simulink model "modelo_experimental"  (R2018a)
settings: Solver=VariableStepAuto  StartTime=0.0  StopTime=1  FixedStep=1e-6  MaxStep=1e-4  RelTol=1e-3
PreLoadFcn:
  | SimulinkInit
InitFcn:
  | SimulinkInit
values from neighbouring files (symbols this model uses):
  C1 = 22e-6    (= 2.2e-05)    [SimulinkInit.m]
  C2 = 22e-6    (= 2.2e-05)    [SimulinkInit.m]
  L1 = 40e-3    (= 0.04)    [SimulinkInit.m]
  L2 = 30e-3    (= 0.03)    [SimulinkInit.m]
  L4 = 315e-3    (= 0.315)    [SimulinkInit.m]
  L5 = 220e-3    (= 0.22)    [SimulinkInit.m]
  L6 = 10e-6    (= 1e-05)    [SimulinkInit.m]
  R1 = 0.1    [SimulinkInit.m]
  R2 = 0.2    [SimulinkInit.m]
  R4 = 5    [SimulinkInit.m]
  R5 = 12    [SimulinkInit.m]
  R6 = 0.001    [SimulinkInit.m]
undefined symbols (not defined in the file or in its folder): Ion, Lithium, sigbuilder_block
libraries: powerlib x48, dsparch4 x12, powerlib_meascontrol x3, electricdrivelib x1
settings Model: Creator=erich  LastModifiedBy=MarioAndres
settings CodeAppCC: StateflowObjectComments=on
settings SimscapeCC: SimscapeNormalizeSystem=off

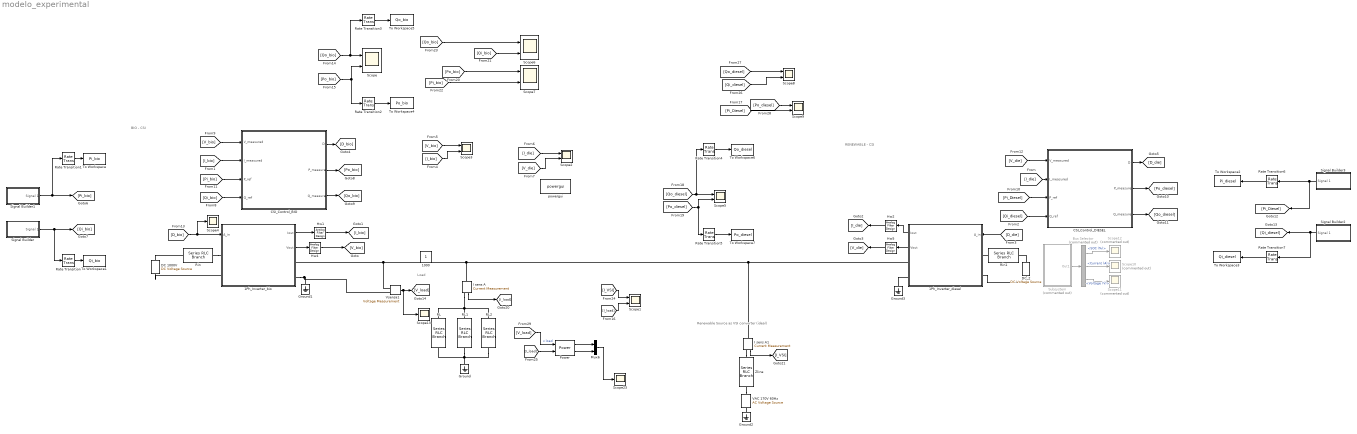
== system modelo_experimental ==
  note: Load
  note: BIO - CSI
  note: RENEWABLE - CSI
  note: Renewable Source as VSI converter (ideal)
  1Ph_Inverter_bio : Subsystem  mask{st_time=0, f_sw=12000, samp_f=1e-6}
      mask prompts: st_time "Tiempo muerto (Start)"; f_sw "Switching frequency"; samp_f "samplig"
      mask Display:
      | port_label('input', 1, 'd', 'texmode', 'on')
      | 
      | port_label('lconn', 1, 'DC +')
      | port_label('lconn', 2, 'DC -')
      | 
      | 
      | port_label('rconn', 1, 'V_{out+}')
      | port_label('rconn', 2, 'B_{out-}')
      | 
      | 
      | port_label('output', 1, 'I_{out}', 'texmode', 'on')
      | port_label('output', 2, 'V_{out}', 'texmode', 'on')
      | 
      | plot([0.1 .9], [0.1 .9])
      | plot([0.2 .4], [.7 .7])
      | plot([0.2 .24], [.65 .65])
      | plot([0.28 .32], [.65 .65])
      | plot([0.36 .40], [.65 .65])
      | 
      | plot([.5:.01:.7], .25+sin(30*[.2:.01:.4])/10)
  1Ph_Inverter_diesel : Subsystem  mask{st_time=0, f_sw=12000, samp_f=1e-6}
      mask prompts: st_time "Tiempo muerto (Start)"; f_sw "Switching frequency"; samp_f "Sampling frequency"
      mask Display:
      | port_label('input', 1, 'd', 'texmode', 'on')
      | 
      | port_label('lconn', 1, 'DC +')
      | port_label('lconn', 2, 'DC -')
      | 
      | 
      | port_label('rconn', 1, 'V_{out+}')
      | port_label('rconn', 2, 'B_{out-}')
      | 
      | 
      | port_label('output', 1, 'I_{out}', 'texmode', 'on')
      | port_label('output', 2, 'V_{out}', 'texmode', 'on')
      | 
      | plot([0.1 .9], [0.1 .9])
      | plot([0.2 .4], [.7 .7])
      | plot([0.2 .24], [.65 .65])
      | plot([0.28 .32], [.65 .65])
      | plot([0.36 .40], [.65 .65])
      | 
      | plot([.5:.01:.7], .25+sin(30*[.2:.01:.4])/10)
  Bus Selector : BusSelector  Commented=on  OutputSignals=SOC (%),Current (A),Voltage (V)
  CSI_Control_BIO : Subsystem  mask{Ki=600, Kp=0.001, wa=60, st_time=1e-3, w0=2*pi*60}
      mask prompts: st_time "Tiempo_muerto"
      mask DialogControl descripcion Prompt: Lazo de control de corriente para inversor monofasico. La entrada es un setpoint de potencia [P, Q]. Con ese setpoint se calcula la referencia de corriente sinusoidal deacuerdo a la tension medida de la red. Por lo anterior este controlador solo es valido para un inversor conectado a la red pues hara que se comporte como un CSI.
  CSI_Control_DIESEL : Subsystem  mask{Ki=600, Kp=0.001, wa=60, st_time=.1, w0=2*pi*60}
      mask prompts: st_time "Tiempo_muerto"
      mask DialogControl descripcion Prompt: Lazo de control de corriente para inversor monofasico. La entrada es un setpoint de potencia [P, Q]. Con ese setpoint se calcula la referencia de corriente sinusoidal deacuerdo a la tension medida de la red. Por lo anterior este controlador solo es valido para un inversor conectado a la red pues hara que se comporte como un CSI.
  DC 1000V : powerlib/Electrical Sources/DC Voltage Source  Amplitude=900  Measurements=None
  DC_2 : powerlib/Electrical Sources/DC Voltage Source  Amplitude=570  Measurements=None
  Ground{,1..3} (4 alike) : powerlib/Elements/Ground  LConnTagsString=a
  Hw{1..2,4..5} (4 alike) : dsparch4/Analog Filter Design  method=Bessel  filttype=Lowpass  N=2  Wlo=7000*2*pi  Whi=80  Rp=2  Rs=80
  I sens A : powerlib/Measurements/Current Measurement  PhasorSimulation=off  OutputType=Complex  PSBequivalent=0
  I sens A1 : powerlib/Measurements/Current Measurement  PhasorSimulation=off  OutputType=Complex  PSBequivalent=0
  Mux6 : Mux  Inputs=2
  Power : powerlib_meascontrol/Measurements/Power  Freq=60  Vinit=[1, 0]  Iinit=[1, 0]  Ts=0
      settings: SourceProductName=Simscape Power Systems
  RL : powerlib/Elements/Series RLC Branch  LConnTagsString=__new0  RConnTagsString=__new0  BranchType=R  Resistance=10  Inductance=500e-3  SetiL0=off  InitialCurrent=0  Capacitance=100e-6  Setx0=off  InitialVoltage=0  Measurements=None
  RL1 : powerlib/Elements/Series RLC Branch  LConnTagsString=__new0  RConnTagsString=__new0  BranchType=RL  Resistance=10  Inductance=5.2  SetiL0=off  InitialCurrent=0  Capacitance=100e-6  Setx0=off  InitialVoltage=0  Measurements=None
  RL2 : powerlib/Elements/Series RLC Branch  LConnTagsString=__new0  RConnTagsString=__new0  BranchType=C  Resistance=30  Inductance=500e-3  SetiL0=off  InitialCurrent=0  Capacitance=2000e-6  Setx0=off  InitialVoltage=0  Measurements=None
  Rate Transition{,1..7} (8 alike) : RateTransition  OutPortSampleTime=1e-4
  Rin : powerlib/Elements/Series RLC Branch  LConnTagsString=__new0  RConnTagsString=__new0  BranchType=R  Resistance=.001  Inductance=0  SetiL0=off  InitialCurrent=0  Capacitance=0  Setx0=off  InitialVoltage=0  Measurements=None
  Rin1 : powerlib/Elements/Series RLC Branch  LConnTagsString=__new0  RConnTagsString=__new0  BranchType=R  Resistance=.001  Inductance=0  SetiL0=off  InitialCurrent=0  Capacitance=0  Setx0=off  InitialVoltage=0  Measurements=None
  Scope{,1..3,5..9} (9 alike) : Scope  NumInputPorts=2
  Scope10 : Scope  Commented=on
  Scope11 : Scope  Commented=on
  Scope12 : Scope  Commented=on
  Scope13 : Scope
  Scope23 : Scope
  Scope4 : Scope
  Signal Builder : Subsystem  Tag=STV Subsys  LoadFcn=sigbuilder_block('load');  StartFcn=sigbuilder_block('start');  StopFcn=sigbuilder_block('stop');  ClipboardFcn=sigbuilder_block('clipboard');  mask(Sigbuilder block){tuvar=[0:10]}
      mask help: Simulink:masks:SigbuilderBlock_MD
      mask init:
      | if ~strcmp(get_param(bdroot(gcbh),'SimulationStatus'),'stopped') tuvar = sigbuilder_block('maskInit'); end
      settings: CopyFcn=sigbuilder_block('copy');  DeleteFcn=sigbuilder_block('delete');  ModelCloseFcn=sigbuilder_block('modelClose');  PreSaveFcn=sigbuilder_block('preSave');  PauseFcn=sigbuilder_block('pause');  ContinueFcn=sigbuilder_block('continue');  NameChangeFcn=sigbuilder_block('namechange');  OpenFcn=sigbuilder_block('open',[0 30 1024.5 488.25 ]);  CloseFcn=sigbuilder_block('close');
      mask Display: plot(0, 0, 100, 100,[2, 2, 32, 32, 2], [68, 8, 8, 68, 68],[32, 2], [38, 38], [32, 19, 2],[53, 60, 44], [32, 17, 17, 2],[16, 16, 31, 31]);txt = getActiveGroup(gcbh);text(2, 100, txt,'verticalAlignment', 'top');
  Signal Builder1 : Subsystem  Tag=STV Subsys  LoadFcn=sigbuilder_block('load');  StartFcn=sigbuilder_block('start');  StopFcn=sigbuilder_block('stop');  ClipboardFcn=sigbuilder_block('clipboard');  mask(Sigbuilder block){tuvar=[0:10]}
      mask help: Simulink:masks:SigbuilderBlock_MD
      mask init:
      | if ~strcmp(get_param(bdroot(gcbh),'SimulationStatus'),'stopped') tuvar = sigbuilder_block('maskInit'); end
      settings: CopyFcn=sigbuilder_block('copy');  DeleteFcn=sigbuilder_block('delete');  ModelCloseFcn=sigbuilder_block('modelClose');  PreSaveFcn=sigbuilder_block('preSave');  PauseFcn=sigbuilder_block('pause');  ContinueFcn=sigbuilder_block('continue');  NameChangeFcn=sigbuilder_block('namechange');  OpenFcn=sigbuilder_block('open',[724.5 348 1024.5 488.25 ]);  CloseFcn=sigbuilder_block('close');
      mask Display: plot(0, 0, 100, 100,[2, 2, 32, 32, 2], [68, 8, 8, 68, 68],[32, 2], [38, 38], [32, 19, 2],[53, 60, 44], [32, 17, 17, 2],[16, 16, 31, 31]);txt = getActiveGroup(gcbh);text(2, 100, txt,'verticalAlignment', 'top');
  Signal Builder2 : Subsystem  Tag=STV Subsys  LoadFcn=sigbuilder_block('load');  StartFcn=sigbuilder_block('start');  StopFcn=sigbuilder_block('stop');  ClipboardFcn=sigbuilder_block('clipboard');  mask(Sigbuilder block){tuvar=[0:10]}
      mask help: Simulink:masks:SigbuilderBlock_MD
      mask init:
      | if ~strcmp(get_param(bdroot(gcbh),'SimulationStatus'),'stopped') tuvar = sigbuilder_block('maskInit'); end
      settings: CopyFcn=sigbuilder_block('copy');  DeleteFcn=sigbuilder_block('delete');  ModelCloseFcn=sigbuilder_block('modelClose');  PreSaveFcn=sigbuilder_block('preSave');  PauseFcn=sigbuilder_block('pause');  ContinueFcn=sigbuilder_block('continue');  NameChangeFcn=sigbuilder_block('namechange');  OpenFcn=sigbuilder_block('open',[0 30 1024.5 488.25 ]);  CloseFcn=sigbuilder_block('close');
      mask Display: plot(0, 0, 100, 100,[2, 2, 32, 32, 2], [68, 8, 8, 68, 68],[32, 2], [38, 38], [32, 19, 2],[53, 60, 44], [32, 17, 17, 2],[16, 16, 31, 31]);txt = getActiveGroup(gcbh);text(2, 100, txt,'verticalAlignment', 'top');
  Signal Builder3 : Subsystem  Tag=STV Subsys  LoadFcn=sigbuilder_block('load');  StartFcn=sigbuilder_block('start');  StopFcn=sigbuilder_block('stop');  ClipboardFcn=sigbuilder_block('clipboard');  mask(Sigbuilder block){tuvar=[0:10]}
      mask help: Simulink:masks:SigbuilderBlock_MD
      mask init:
      | if ~strcmp(get_param(bdroot(gcbh),'SimulationStatus'),'stopped') tuvar = sigbuilder_block('maskInit'); end
      settings: CopyFcn=sigbuilder_block('copy');  DeleteFcn=sigbuilder_block('delete');  ModelCloseFcn=sigbuilder_block('modelClose');  PreSaveFcn=sigbuilder_block('preSave');  PauseFcn=sigbuilder_block('pause');  ContinueFcn=sigbuilder_block('continue');  NameChangeFcn=sigbuilder_block('namechange');  OpenFcn=sigbuilder_block('open',[6 30 1012.5 447.75 ]);  CloseFcn=sigbuilder_block('close');
      mask Display: plot(0, 0, 100, 100,[2, 2, 32, 32, 2], [68, 8, 8, 68, 68],[32, 2], [38, 38], [32, 19, 2],[53, 60, 44], [32, 17, 17, 2],[16, 16, 31, 31]);txt = getActiveGroup(gcbh);text(2, 100, txt,'verticalAlignment', 'top');
  Subsystem : Subsystem  Commented=on
  To Workspace : ToWorkspace  VariableName=Pi_bio  SaveFormat=Timeseries  SampleTime=-1
  To Workspace1 : ToWorkspace  VariableName=Qi_bio  SaveFormat=Timeseries  SampleTime=-1
  To Workspace2 : ToWorkspace  VariableName=Pi_diesel  SaveFormat=Timeseries  SampleTime=-1
  To Workspace3 : ToWorkspace  VariableName=Qi_diesel  SaveFormat=Timeseries  SampleTime=-1
  To Workspace4 : ToWorkspace  VariableName=Po_bio  SaveFormat=Timeseries  SampleTime=-1
  To Workspace5 : ToWorkspace  VariableName=Qo_bio  SaveFormat=Timeseries  SampleTime=-1
  To Workspace6 : ToWorkspace  VariableName=Qo_diesel  SaveFormat=Timeseries  SampleTime=-1
  To Workspace7 : ToWorkspace  VariableName=Po_diesel  SaveFormat=Timeseries  SampleTime=-1
  VAC 170V 60Hz : powerlib/Electrical Sources/AC Voltage Source  Amplitude=170  Phase=0  Frequency=60  SampleTime=0  Measurements=None  BusType=swing  Pref=10e3  Qref=0  Qmin=-inf  Qmax=+inf
  Vsensa1 : powerlib/Measurements/Voltage Measurement  PhasorSimulation=off  OutputType=Complex  PSBequivalent=0
  Zline : powerlib/Elements/Series RLC Branch  LConnTagsString=__new0  RConnTagsString=__new0  BranchType=RL  Resistance=R6  Inductance=L6  SetiL0=off  InitialCurrent=0  Capacitance=100e-6  Setx0=off  InitialVoltage=0  Measurements=None
  powergui : powerlib/powergui  Priority=1  SimulationMode=Continuous  SampleTime=50e-6  frequency=60  Iterations=50  frequencyindice=0  Pbase=100e6  ErrMax=1e-4  UnitsV=kV  UnitsW=MW  buscounter=0  FunctionMessages=off  echomessages=off  EnableUseOfTLC=off  CurrentSourceSwitches=off  DisableSnubberDevices=off  DisableRonSwitches=off  DisableVfSwitches=off  DisplayEquations=off  SolverType=Tustin/Backward Euler (TBE)  Interpol=off  ExternalGateDelay=off  methode=off  Ts=100  x0status=blocks  SPID=on  SwTol=0  HookPort=off  RestoreLinks=warning  ResistiveCurrentMeasurement=off  Frange=[0:2:500]  Ylog=off  Xlog=on  ShowGrid=off  save=off  variable=ZData  structure=0  ZoomFFT=off  StartTime=0.0  cycles=1  DisplayStyle=1  fundamental=60  FreqAxis=off  MaxFrequency=1000  frequencyindicesteady=1  RmsSteady=1  display=off
  1000 : Constant  IOType=siggen
  wires:
  [D_bio] -> Scope4/1, 1Ph_Inverter_bio/1(A_in)
  [D_die] -> 1Ph_Inverter_diesel/1(A_in)
  [I_bio] -> Scope3/2
  [V_bio] -> Scope3/1
  [I_die] -> Scope2/1
  [V_die] -> Scope2/2
  1Ph_Inverter_bio/2(Vout) -> Hw4/1
  1Ph_Inverter_diesel/2(Vout) -> Hw5/1
  1Ph_Inverter_bio/1(Iout) -> Hw1/1
  1Ph_Inverter_diesel/1(Iout) -> Hw2/1
  I sens A/1 -> [I_load]
  Bus Selector/2 -> Scope10/1  "<Current (A)>"
  Bus Selector/1 -> Scope12/1  "<SOC (%)>"
  Bus Selector/3 -> Scope11/1  "<Voltage (V)>"
  Subsystem/1(Out1) -> Bus Selector/1
  Power/2 -> Mux6/2
  [I_load] -> Power/2
  Mux6/1 -> Scope23/1
  [V_load] -> Power/1  "v load"
  Power/1 -> Mux6/1
  I sens A1/1 -> [I_VSI]
  Rate Transition1/1 -> To Workspace/1
  Rate Transition/1 -> To Workspace1/1
  Signal Builder/1(Signal 1) -> Rate Transition/1, [Qi_bio]
  Signal Builder1/1(Signal 1) -> Rate Transition1/1, [Pi_bio]
  [Qo_bio] -> Rate Transition3/1, Scope/1
  Rate Transition3/1 -> To Workspace5/1
  Rate Transition2/1 -> To Workspace4/1
  [Po_bio] -> Scope/2, Rate Transition2/1
  Signal Builder3/1(Signal 1) -> [Pi_Diesel], Rate Transition6/1
  Rate Transition6/1 -> To Workspace2/1
  Signal Builder2/1(Signal 1) -> [Qi_diesel], Rate Transition7/1
  Rate Transition7/1 -> To Workspace3/1
  Rate Transition4/1 -> To Workspace6/1
  [Po_diesel] -> Rate Transition5/1, Scope5/2
  [Qo_diesel] -> Rate Transition4/1, Scope5/1
  Rate Transition5/1 -> To Workspace7/1
  [Pi_bio] -> CSI_Control_BIO/3(P_ref)
  [Qi_bio] -> CSI_Control_BIO/4(Q_ref)
  CSI_Control_BIO/2(P_measure) -> [Po_bio]
  CSI_Control_BIO/1(D) -> [D_bio]
  CSI_Control_BIO/3(Q_measure) -> [Qo_bio]
  [V_bio] -> CSI_Control_BIO/1(V_measured)
  [I_bio] -> CSI_Control_BIO/2(I_measured)
  [Pi_Diesel] -> CSI_Control_DIESEL/3(P_ref)
  [V_die] -> CSI_Control_DIESEL/1(V_measured)
  CSI_Control_DIESEL/1(D) -> [D_die]
  CSI_Control_DIESEL/3(Q_measure) -> [Qo_diesel]
  [I_die] -> CSI_Control_DIESEL/2(I_measured)
  CSI_Control_DIESEL/2(P_measure) -> [Po_diesel]
  [Qi_diesel] -> CSI_Control_DIESEL/4(Q_ref)
  [Qo_diesel] -> Scope8/1
  [Qi_diesel] -> Scope8/2
  [Po_diesel] -> Scope9/1
  [Pi_Diesel] -> Scope9/2
  [Pi_bio] -> Scope7/2
  [Qo_bio] -> Scope6/1
  [Qi_bio] -> Scope6/2
  [Po_bio] -> Scope7/1
  Hw1/1 -> [I_bio]
  Hw4/1 -> [V_bio]
  Hw2/1 -> [I_die]
  Hw5/1 -> [V_die]
  [I_VSI] -> Scope1/1
  [I_load] -> Scope1/2
  Vsensa1/1 -> Scope13/1, [V_load]
  connections:
  RL/LConn1 -- I sens A/RConn1 -- RL2/LConn1 -- RL1/LConn1
  Ground/LConn1 -- RL1/RConn1 -- RL2/RConn1 -- RL/RConn1
  1Ph_Inverter_bio/RConn2 -- Vsensa1/LConn2 -- Ground1/LConn1
  Rin/RConn1 -- 1Ph_Inverter_bio/LConn1
  1Ph_Inverter_diesel/RConn2 -- Ground3/LConn1
  I sens A/LConn1 -- Vsensa1/LConn1 -- 1Ph_Inverter_bio/RConn1 -- I sens A1/LConn1 -- 1Ph_Inverter_diesel/RConn1
  Zline/RConn1 -- VAC 170V 60Hz/RConn1
  Ground2/LConn1 -- VAC 170V 60Hz/LConn1
  I sens A1/RConn1 -- Zline/LConn1
  DC 1000V/RConn1 -- Rin/LConn1
  DC 1000V/LConn1 -- 1Ph_Inverter_bio/LConn2
  DC_2/RConn1 -- Rin1/LConn1
  1Ph_Inverter_diesel/LConn2 -- DC_2/LConn1
  Rin1/RConn1 -- 1Ph_Inverter_diesel/LConn1

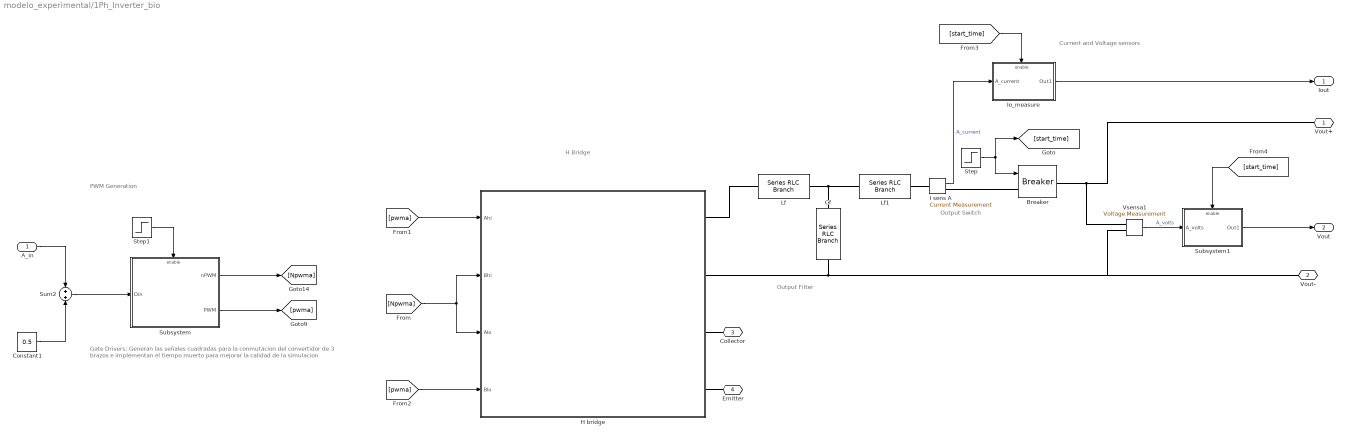
== system modelo_experimental/1Ph_Inverter_bio ==
  note: PWM Generation
  note: H Bridge
  note: Output Filter
  note: Current and Voltage sensors
  note: Output Switch
  note: Gate Drivers: Generan las señales cuadradas para
      | la conmutacion del convertidor de 3 brazos e implementan el
      | tiempo muerto para mejorar la calidad de la simulacion
  A_in : Inport
  Breaker : powerlib/Elements/Breaker  InitialState=0  SwitchingTimes="[1/60  5/60]"  External=on  BreakerResistance=0.01  SnubberResistance=1e6  SnubberCapacitance=inf  Measurements=None  MoreParameters=on  NoBreakLoop=off
      settings: SourceProductName=Simscape Power Systems
  Cf : powerlib/Elements/Series RLC Branch  LConnTagsString=__new0  RConnTagsString=__new0  BranchType=C  Resistance=1  Inductance=1e-3  SetiL0=off  InitialCurrent=0  Capacitance=C1  Setx0=off  InitialVoltage=0  Measurements=None
  Constant1 : Constant  Value=0.5
  H bridge : Subsystem
      mask Display:
      | port_label('input', 1, '\fontsize{12} Ahi', 'texmode', 'on')
      | port_label('input', 2, '\fontsize{12} Alo', 'texmode', 'on')
      | port_label('input', 3, '\fontsize{12} Bhi', 'texmode', 'on')
      | port_label('input', 4, '\fontsize{12} Blo', 'texmode', 'on')
      | 
      | 
      | port_label('rconn', 1, '\fontsize{12} V_{out} +', 'texmode', 'on')
      | port_label('rconn', 2, '\fontsize{12} V_{out} -', 'texmode', 'on')
      | 
      | port_label('rconn', 3, '\fontsize{12} Collector', 'texmode', 'on')
      | port_label('rconn', 4, '\fontsize{12} Emitter', 'texmode', 'on')
      | 
      | lvx = [.1 .1];
      | lvy = [.1 .2];
      | lhx = [.1 .2];
      | lhy = [.1 .1];
      | 
      | 
      | % se dibujan los interruptores de la izquierda
      | plot(lvx+.07, lvy*.8+.028+.1)
      | plot(lvx+.1, lvy+.1)
      | plot(lhx*.5+.15, lhy+.1)
      | plot(lhx*.5+.15, lhy+.2)
      | plot(lhx*.5+.07, lhy+.15)
      | 
      | d=0.5;
      | 
      | plot(lvx+.07, lvy*.8+.028+.1+d)
      | plot(lvx+.1, lvy+.1+d)
      | plot(lhx*.5+.15, lhy+.1+d)
      | plot(lhx*.5+.15, lhy+.2+d)
      | plot(lhx*.5+.07, lhy+.15+d)
      | 
      | 
      | % se dibujan los interruptores del medio
      | h=.3;
      | 
      | %plot(lvx+.07+h, lvy*.8+.028+.1)
      | %plot(lvx+.1+h, lvy+.1)
      | %plot(lhx*.5+.15+h, lhy+.1)
      | %plot(lhx*.5+.15+h, lhy+.2)
      | %plot(lhx*.5+.07+h, lhy+.15)
      | 
      | %plot(lvx+.07+h, lvy*.8+.028+.1+d)
      | %plot(lvx+.1+h, lvy+.1+d)
      | %plot(lhx*.5+.15+h, lhy+.1+d)
      | %plot(lhx*.5+.15+h, lhy+.2+d)
      | %plot(lhx*.5+.07+h, lhy+.15+d)
      | 
      | % se dibujan los interruptores de la derecha
      | h=.6
      | 
      | plot(lvx+.07+h, lvy*.8+.028+.1)
      | plot(lvx+.1+h, lvy+.1)
      | plot(lhx*.5+.15+h, lhy+.1)
      | plot(lhx*.5+.15+h, lhy+.2)
      | plot(lhx*.5+.07+h, lhy+.15)
      | 
      | plot(lvx+.07+h, lvy*.8+.028+.1+d)
      | plot(lvx+.1+h, lvy+.1+d)
      | plot(lhx*.5+.15+h, lhy+.1+d)
      | plot(lhx*.5+.15+h, lhy+.2+d)
      | plot(lhx*.5+.07+h, lhy+.15+d)
      | 
      | 
      | % se conectan los interruptores.
      | plot(lvx+.15, lvy*4-.1)
      | %plot(lvx+.15+.3, lvy*4-.1)
      | plot(lvx+.15+.6, lvy*4-.1)
      | 
      | 
      | plot(lvx+.15, lvy+.7)
      | %plot(lvx+.15+.3, lvy+.7)
      | plot(lvx+.15+.6, lvy+.7)
      | 
      | plot(lvx+.15, lvy)
      | %plot(lvx+.15+.3, lvy)
      | plot(lvx+.15+.6, lvy)
      | 
      | plot(lhx*6-.35, lhy)
      | plot(lhx*6-.35, lhy+.8)
      | 
      | % raul esteban alzate 313 515 86 11
  I sens A : powerlib/Measurements/Current Measurement  PhasorSimulation=off  OutputType=Complex  PSBequivalent=0
  Io_measure : Subsystem
  Lf : powerlib/Elements/Series RLC Branch  LConnTagsString=__new0  RConnTagsString=__new0  BranchType=RL  Resistance=R1  Inductance=L1  SetiL0=off  InitialCurrent=0  Capacitance=1e-6  Setx0=off  InitialVoltage=0  Measurements=None
  Lf1 : powerlib/Elements/Series RLC Branch  LConnTagsString=__new0  RConnTagsString=__new0  BranchType=RL  Resistance=R4  Inductance=L4  SetiL0=off  InitialCurrent=0  Capacitance=1e-6  Setx0=off  InitialVoltage=0  Measurements=None
  Step : Step  Time=st_time  SampleTime=0
  Step1 : Step  Time=st_time  SampleTime=0
  Subsystem : Subsystem
  Subsystem1 : Subsystem
  Sum2 : Sum
  Vsensa1 : powerlib/Measurements/Voltage Measurement  PhasorSimulation=off  OutputType=Complex  PSBequivalent=0
  Vout+ : PMIOPort  Side=Right
  Vout- : PMIOPort  Port=2  Side=Right
  Collector : PMIOPort  Port=3  Side=Left
  Emitter : PMIOPort  Port=4  Side=Left
  Iout : Outport
  Vout : Outport  Port=2
  wires:
  Constant1/1 -> Sum2/2
  A_in/1 -> Sum2/1
  [pwma] -> H bridge/1(Ahi)
  [Npwma] -> H bridge/2(Bhi), H bridge/3(Alo)
  [pwma] -> H bridge/4(Blo)
  Step/1 -> [start_time], Breaker/1
  Sum2/1 -> Subsystem/1(Din)
  Subsystem/1(nPWM) -> [Npwma]
  Subsystem/2(PWM) -> [pwma]
  Step1/1 -> Subsystem/Enable
  I sens A/1 -> Io_measure/1(A_current)  "A_current"
  Io_measure/1(Out1) -> Iout/1
  [start_time] -> Io_measure/Enable
  Vsensa1/1 -> Subsystem1/1(A_volts)  "A_volts"
  Subsystem1/1(Out1) -> Vout/1
  [start_time] -> Subsystem1/Enable
  connections:
  H bridge/RConn3 -- Collector/RConn1
  H bridge/RConn4 -- Emitter/RConn1
  Lf/LConn1 -- H bridge/RConn1
  H bridge/RConn2 -- Vsensa1/LConn2 -- Vout-/RConn1 -- Cf/RConn1
  Breaker/LConn1 -- I sens A/RConn1
  Breaker/RConn1 -- Vsensa1/LConn1 -- Vout+/RConn1
  Lf1/RConn1 -- I sens A/LConn1
  Cf/LConn1 -- Lf1/LConn1 -- Lf/RConn1

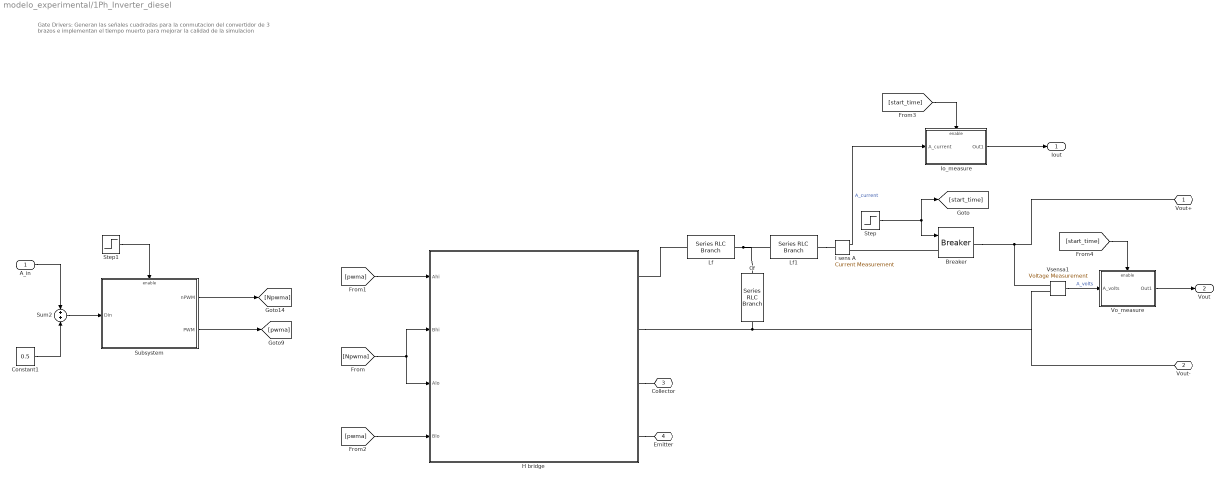
== system modelo_experimental/1Ph_Inverter_diesel ==
  note: Gate Drivers: Generan las señales cuadradas para
      | la conmutacion del convertidor de 3 brazos e implementan el
      | tiempo muerto para mejorar la calidad de la simulacion
  A_in : Inport
  Breaker : powerlib/Elements/Breaker  InitialState=0  SwitchingTimes="[1/60  5/60]"  External=on  BreakerResistance=0.01  SnubberResistance=1e6  SnubberCapacitance=inf  Measurements=None  MoreParameters=on  NoBreakLoop=off
      settings: SourceProductName=Simscape Power Systems
  Cf : powerlib/Elements/Series RLC Branch  LConnTagsString=__new0  RConnTagsString=__new0  BranchType=C  Resistance=1  Inductance=1e-3  SetiL0=off  InitialCurrent=0  Capacitance=C2  Setx0=off  InitialVoltage=0  Measurements=None
  Constant1 : Constant  Value=0.5
  H bridge : Subsystem
      mask Display:
      | port_label('input', 1, '\fontsize{12} Ahi', 'texmode', 'on')
      | port_label('input', 2, '\fontsize{12} Alo', 'texmode', 'on')
      | port_label('input', 3, '\fontsize{12} Bhi', 'texmode', 'on')
      | port_label('input', 4, '\fontsize{12} Blo', 'texmode', 'on')
      | 
      | 
      | port_label('rconn', 1, '\fontsize{12} V_{out} +', 'texmode', 'on')
      | port_label('rconn', 2, '\fontsize{12} V_{out} -', 'texmode', 'on')
      | 
      | port_label('rconn', 3, '\fontsize{12} Collector', 'texmode', 'on')
      | port_label('rconn', 4, '\fontsize{12} Emitter', 'texmode', 'on')
      | 
      | lvx = [.1 .1];
      | lvy = [.1 .2];
      | lhx = [.1 .2];
      | lhy = [.1 .1];
      | 
      | 
      | % se dibujan los interruptores de la izquierda
      | plot(lvx+.07, lvy*.8+.028+.1)
      | plot(lvx+.1, lvy+.1)
      | plot(lhx*.5+.15, lhy+.1)
      | plot(lhx*.5+.15, lhy+.2)
      | plot(lhx*.5+.07, lhy+.15)
      | 
      | d=0.5;
      | 
      | plot(lvx+.07, lvy*.8+.028+.1+d)
      | plot(lvx+.1, lvy+.1+d)
      | plot(lhx*.5+.15, lhy+.1+d)
      | plot(lhx*.5+.15, lhy+.2+d)
      | plot(lhx*.5+.07, lhy+.15+d)
      | 
      | 
      | % se dibujan los interruptores del medio
      | h=.3;
      | 
      | %plot(lvx+.07+h, lvy*.8+.028+.1)
      | %plot(lvx+.1+h, lvy+.1)
      | %plot(lhx*.5+.15+h, lhy+.1)
      | %plot(lhx*.5+.15+h, lhy+.2)
      | %plot(lhx*.5+.07+h, lhy+.15)
      | 
      | %plot(lvx+.07+h, lvy*.8+.028+.1+d)
      | %plot(lvx+.1+h, lvy+.1+d)
      | %plot(lhx*.5+.15+h, lhy+.1+d)
      | %plot(lhx*.5+.15+h, lhy+.2+d)
      | %plot(lhx*.5+.07+h, lhy+.15+d)
      | 
      | % se dibujan los interruptores de la derecha
      | h=.6
      | 
      | plot(lvx+.07+h, lvy*.8+.028+.1)
      | plot(lvx+.1+h, lvy+.1)
      | plot(lhx*.5+.15+h, lhy+.1)
      | plot(lhx*.5+.15+h, lhy+.2)
      | plot(lhx*.5+.07+h, lhy+.15)
      | 
      | plot(lvx+.07+h, lvy*.8+.028+.1+d)
      | plot(lvx+.1+h, lvy+.1+d)
      | plot(lhx*.5+.15+h, lhy+.1+d)
      | plot(lhx*.5+.15+h, lhy+.2+d)
      | plot(lhx*.5+.07+h, lhy+.15+d)
      | 
      | 
      | % se conectan los interruptores.
      | plot(lvx+.15, lvy*4-.1)
      | %plot(lvx+.15+.3, lvy*4-.1)
      | plot(lvx+.15+.6, lvy*4-.1)
      | 
      | 
      | plot(lvx+.15, lvy+.7)
      | %plot(lvx+.15+.3, lvy+.7)
      | plot(lvx+.15+.6, lvy+.7)
      | 
      | plot(lvx+.15, lvy)
      | %plot(lvx+.15+.3, lvy)
      | plot(lvx+.15+.6, lvy)
      | 
      | plot(lhx*6-.35, lhy)
      | plot(lhx*6-.35, lhy+.8)
      | 
      | % raul esteban alzate 313 515 86 11
  I sens A : powerlib/Measurements/Current Measurement  PhasorSimulation=off  OutputType=Complex  PSBequivalent=0
  Io_measure : Subsystem
  Lf : powerlib/Elements/Series RLC Branch  LConnTagsString=__new0  RConnTagsString=__new0  BranchType=RL  Resistance=R2  Inductance=L2  SetiL0=off  InitialCurrent=0  Capacitance=1e-6  Setx0=off  InitialVoltage=0  Measurements=None
  Lf1 : powerlib/Elements/Series RLC Branch  LConnTagsString=__new0  RConnTagsString=__new0  BranchType=RL  Resistance=R5  Inductance=L5  SetiL0=off  InitialCurrent=0  Capacitance=1e-6  Setx0=off  InitialVoltage=0  Measurements=None
  Step : Step  Time=st_time  SampleTime=0
  Step1 : Step  Time=st_time  SampleTime=0
  Subsystem : Subsystem
  Sum2 : Sum
  Vo_measure : Subsystem
  Vsensa1 : powerlib/Measurements/Voltage Measurement  PhasorSimulation=off  OutputType=Complex  PSBequivalent=0
  Vout+ : PMIOPort  Side=Right
  Vout- : PMIOPort  Port=2  Side=Right
  Collector : PMIOPort  Port=3  Side=Left
  Emitter : PMIOPort  Port=4  Side=Left
  Iout : Outport
  Vout : Outport  Port=2
  wires:
  [pwma] -> H bridge/4(Blo)
  [Npwma] -> H bridge/3(Alo), H bridge/2(Bhi)
  [pwma] -> H bridge/1(Ahi)
  A_in/1 -> Sum2/1
  Constant1/1 -> Sum2/2
  Step/1 -> [start_time], Breaker/1
  Sum2/1 -> Subsystem/1(Din)
  Subsystem/1(nPWM) -> [Npwma]
  Subsystem/2(PWM) -> [pwma]
  Step1/1 -> Subsystem/Enable
  Vsensa1/1 -> Vo_measure/1(A_volts)  "A_volts"
  Vo_measure/1(Out1) -> Vout/1
  I sens A/1 -> Io_measure/1(A_current)  "A_current"
  Io_measure/1(Out1) -> Iout/1
  [start_time] -> Io_measure/Enable
  [start_time] -> Vo_measure/Enable
  connections:
  Cf/RConn1 -- Vsensa1/LConn2 -- Vout-/RConn1 -- H bridge/RConn2
  Lf/LConn1 -- H bridge/RConn1
  H bridge/RConn4 -- Emitter/RConn1
  H bridge/RConn3 -- Collector/RConn1
  Breaker/LConn1 -- I sens A/RConn1
  Breaker/RConn1 -- Vsensa1/LConn1 -- Vout+/RConn1
  Lf/RConn1 -- Cf/LConn1 -- Lf1/LConn1
  Lf1/RConn1 -- I sens A/LConn1

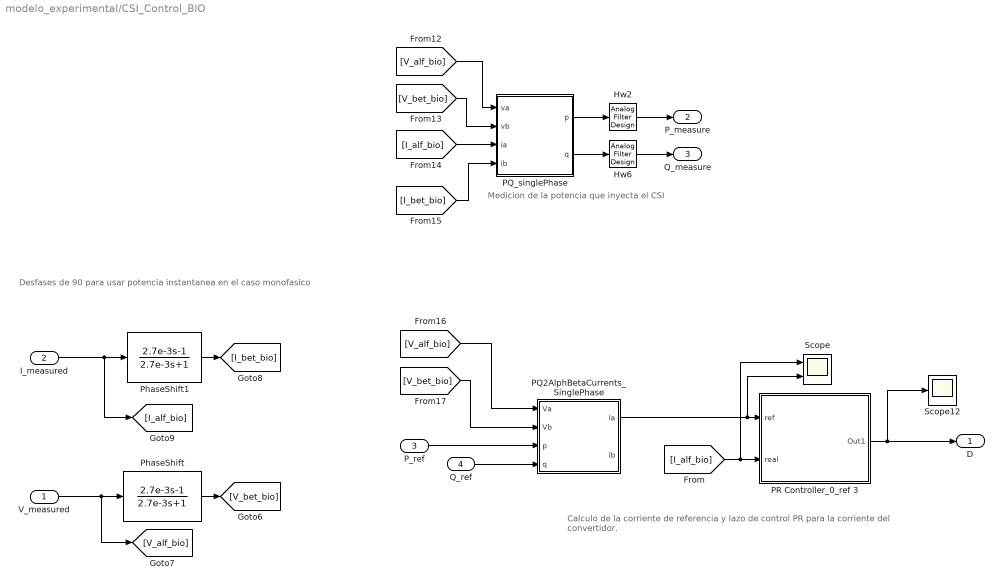
== system modelo_experimental/CSI_Control_BIO ==
  note: Medicion de la potencia que inyecta el CSI
  note: Desfases de 90 para usar potencia
      | instantanea en el caso monofasico
  note: Calculo de la corriente de referencia
      | y lazo de control PR para la corriente
      | del convertidor.
  V_measured : Inport
  I_measured : Inport  Port=2
  P_ref : Inport  Port=3
  Q_ref : Inport  Port=4
  Hw2 : dsparch4/Analog Filter Design  method=Bessel  filttype=Lowpass  N=4  Wlo=30*2*pi  Whi=80  Rp=2  Rs=80
  Hw6 : dsparch4/Analog Filter Design  method=Bessel  filttype=Lowpass  N=4  Wlo=30*2*pi  Whi=80  Rp=2  Rs=80
  PQ2AlphBetaCurrents_SinglePhase : MATLAB Function  TreatAsAtomicUnit=on
  PQ_singlePhase : MATLAB Function  TreatAsAtomicUnit=on
  PR Controller_0_ref 3 : Subsystem  mask{Kp=Kp, Ki=Ki, wa=wa, w0=w0, st_time=st_time}
      mask prompts: Kp "Ganancia Proporcional"; Ki "Ganancia Integral"; wa "Ancho camapana resonancia"; w0 "Frecuencia Central"; st_time "Tiempo muerto (Start)"
      mask Display:
      | port_label('input',1,'ref')
      | port_label('input',2,'sens')
      | port_label('output',1,'out')
      | 
      | plot(.4+[0:.01:pi/10], .32+sin(40*[0:.01:pi/10])/13)
      | 
      | plot([.4 .6],.05+[.5 .7])
      | plot([.4 .6],.05+[.9 .7])
      | plot([.4 .4],.05+[.9 .5])
      | 
      | text(.27,.37,'\fontsize{25} \int', 'texmode', 'on')
  PhaseShift : TransferFcn  Numerator=[2.7e-3 -1]  Denominator=[2.7e-3 1]
  PhaseShift1 : TransferFcn  Numerator=[2.7e-3 -1]  Denominator=[2.7e-3 1]
  Scope : Scope  NumInputPorts=2
  Scope12 : Scope
  D : Outport
  P_measure : Outport  Port=2
  Q_measure : Outport  Port=3
  wires:
  PQ_singlePhase/2(q) -> Hw6/1
  PQ2AlphBetaCurrents_SinglePhase/1(Ia) -> Scope/2, PR Controller_0_ref 3/1(ref)
  PR Controller_0_ref 3/1(Out1) -> D/1, Scope12/1
  [I_bet_bio] -> PQ_singlePhase/4(ib)
  [I_alf_bio] -> Scope/1, PR Controller_0_ref 3/2(real)
  I_measured/1 -> [I_alf_bio], PhaseShift1/1
  [V_bet_bio] -> PQ2AlphBetaCurrents_SinglePhase/2(Vb)
  Hw6/1 -> Q_measure/1
  P_ref/1 -> PQ2AlphBetaCurrents_SinglePhase/3(p)
  Q_ref/1 -> PQ2AlphBetaCurrents_SinglePhase/4(q)
  PhaseShift/1 -> [V_bet_bio]
  PQ_singlePhase/1(p) -> Hw2/1
  [V_alf_bio] -> PQ_singlePhase/1(va)
  [I_alf_bio] -> PQ_singlePhase/3(ia)
  Hw2/1 -> P_measure/1
  [V_alf_bio] -> PQ2AlphBetaCurrents_SinglePhase/1(Va)
  PhaseShift1/1 -> [I_bet_bio]
  V_measured/1 -> [V_alf_bio], PhaseShift/1
  [V_bet_bio] -> PQ_singlePhase/2(vb)

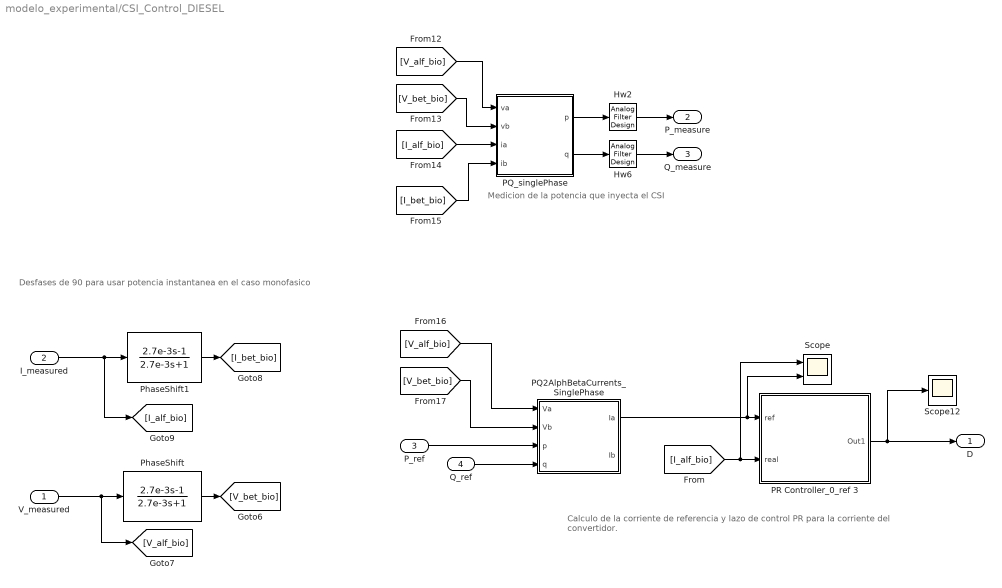
== system modelo_experimental/CSI_Control_DIESEL ==
  note: Calculo de la corriente de referencia
      | y lazo de control PR para la corriente
      | del convertidor.
  note: Desfases de 90 para usar potencia
      | instantanea en el caso monofasico
  note: Medicion de la potencia que inyecta el CSI
  V_measured : Inport
  I_measured : Inport  Port=2
  P_ref : Inport  Port=3
  Q_ref : Inport  Port=4
  Hw2 : dsparch4/Analog Filter Design  method=Bessel  filttype=Lowpass  N=4  Wlo=30*2*pi  Whi=80  Rp=2  Rs=80
  Hw6 : dsparch4/Analog Filter Design  method=Bessel  filttype=Lowpass  N=4  Wlo=30*2*pi  Whi=80  Rp=2  Rs=80
  PQ2AlphBetaCurrents_SinglePhase : MATLAB Function  TreatAsAtomicUnit=on
  PQ_singlePhase : MATLAB Function  TreatAsAtomicUnit=on
  PR Controller_0_ref 3 : Subsystem  mask{Kp=Kp, Ki=Ki, wa=wa, w0=w0, st_time=st_time}
      mask prompts: Kp "Ganancia Proporcional"; Ki "Ganancia Integral"; wa "Ancho camapana resonancia"; w0 "Frecuencia Central"; st_time "Tiempo muerto (Start)"
      mask Display:
      | port_label('input',1,'ref')
      | port_label('input',2,'sens')
      | port_label('output',1,'out')
      | 
      | plot(.4+[0:.01:pi/10], .32+sin(40*[0:.01:pi/10])/13)
      | 
      | plot([.4 .6],.05+[.5 .7])
      | plot([.4 .6],.05+[.9 .7])
      | plot([.4 .4],.05+[.9 .5])
      | 
      | text(.27,.37,'\fontsize{25} \int', 'texmode', 'on')
  PhaseShift : TransferFcn  Numerator=[2.7e-3 -1]  Denominator=[2.7e-3 1]
  PhaseShift1 : TransferFcn  Numerator=[2.7e-3 -1]  Denominator=[2.7e-3 1]
  Scope : Scope  NumInputPorts=2
  Scope12 : Scope
  D : Outport
  P_measure : Outport  Port=2
  Q_measure : Outport  Port=3
  wires:
  [V_bet_bio] -> PQ_singlePhase/2(vb)
  V_measured/1 -> PhaseShift/1, [V_alf_bio]
  PhaseShift1/1 -> [I_bet_bio]
  [V_alf_bio] -> PQ2AlphBetaCurrents_SinglePhase/1(Va)
  Hw2/1 -> P_measure/1
  [I_alf_bio] -> PQ_singlePhase/3(ia)
  [V_alf_bio] -> PQ_singlePhase/1(va)
  PQ_singlePhase/1(p) -> Hw2/1
  PhaseShift/1 -> [V_bet_bio]
  Q_ref/1 -> PQ2AlphBetaCurrents_SinglePhase/4(q)
  P_ref/1 -> PQ2AlphBetaCurrents_SinglePhase/3(p)
  Hw6/1 -> Q_measure/1
  [V_bet_bio] -> PQ2AlphBetaCurrents_SinglePhase/2(Vb)
  I_measured/1 -> PhaseShift1/1, [I_alf_bio]
  [I_alf_bio] -> PR Controller_0_ref 3/2(real), Scope/1
  [I_bet_bio] -> PQ_singlePhase/4(ib)
  PR Controller_0_ref 3/1(Out1) -> Scope12/1, D/1
  PQ2AlphBetaCurrents_SinglePhase/1(Ia) -> PR Controller_0_ref 3/1(ref), Scope/2
  PQ_singlePhase/2(q) -> Hw6/1

== system modelo_experimental/Signal Builder ==
  Demux : Demux  Tag=STV Demux  Outputs=1
  FromWs : FromWorkspace  Tag=STV FromWs  VariableName=tuvar  SampleTime=0
      SigBuilderData=|
      | common.afterFinalStr = 'Extrapolate'
      | common.sampleTime = 0
      | dataSet.timeRange = [0 10]
      | dataSet.name = 'Group 1'
      | sbobj.Groups.Name = 'Group 1'
      | sbobj.Groups.Signals.Name = 'Signal 1'
      | sbobj.Groups.Signals.XData = [0 0.1 0.1 0.2 0.2 0.3 0.3 0.4 0.4 0.5 0.5 0.6 0.6 0.7 0.7 0.8 0.8 0.9 0.9 10]
      | sbobj.Groups.Signals.YData = [0 0 500 500 1000 1000 1500 1500 2000 2000 2500 2500 3000 3000 3500 3500 4000 4000 4500 4500]
  Signal 1 : Outport  Tag=STV Outport
  wires:
  Demux/1 -> Signal 1/1
  FromWs/1 -> Demux/1

== system modelo_experimental/Signal Builder1 ==
  Demux : Demux  Tag=STV Demux  Outputs=1
  FromWs : FromWorkspace  Tag=STV FromWs  VariableName=tuvar  SampleTime=0
      SigBuilderData=|
      | common.afterFinalStr = 'Extrapolate'
      | common.sampleTime = 0
      | dataSet.timeRange = [0 10]
      | dataSet.name = 'Group 1'
      | sbobj.Groups.Name = 'Group 1'
      | sbobj.Groups.Signals.Name = 'Signal 1'
      | sbobj.Groups.Signals.XData = [0 0.1 0.1 0.4 0.4 0.8 0.8 10]
      | sbobj.Groups.Signals.YData = [0 0 100 100 200 200 500 500]
  Signal 1 : Outport  Tag=STV Outport
  wires:
  FromWs/1 -> Demux/1
  Demux/1 -> Signal 1/1

== system modelo_experimental/Signal Builder2 ==
  Demux : Demux  Tag=STV Demux  Outputs=1
  FromWs : FromWorkspace  Tag=STV FromWs  VariableName=tuvar  SampleTime=0
      SigBuilderData=|
      | common.afterFinalStr = 'Extrapolate'
      | common.sampleTime = 0
      | dataSet.timeRange = [0 10]
      | dataSet.name = 'Group 1'
      | sbobj.Groups.Name = 'Group 1'
      | sbobj.Groups.Signals.Name = 'Signal 1'
      | sbobj.Groups.Signals.XData = [0 0.1 0.1 0.2 0.2 0.3 0.3 0.4 0.4 0.5 0.5 0.6 0.6 0.7 0.7 0.8 0.8 0.9 0.9 10]
      | sbobj.Groups.Signals.YData = [0 0 500 500 1000 1000 1500 1500 2000 2000 2500 2500 3000 3000 3500 3500 4000 4000 4500 4500]
  Signal 1 : Outport  Tag=STV Outport
  wires:
  FromWs/1 -> Demux/1
  Demux/1 -> Signal 1/1

== system modelo_experimental/Signal Builder3 ==
  Demux : Demux  Tag=STV Demux  Outputs=1
  FromWs : FromWorkspace  Tag=STV FromWs  VariableName=tuvar  SampleTime=0
      SigBuilderData=|
      | common.afterFinalStr = 'Extrapolate'
      | common.sampleTime = 0
      | dataSet.timeRange = [0 10]
      | dataSet.name = 'Group 1'
      | sbobj.Groups.Name = 'Group 1'
      | sbobj.Groups.Signals.Name = 'Signal 1'
      | sbobj.Groups.Signals.XData = [0 0.1 0.1 0.4 0.4 0.8 0.8 10]
      | sbobj.Groups.Signals.YData = [0 0 100 100 200 200 500 500]
  Signal 1 : Outport  Tag=STV Outport
  wires:
  Demux/1 -> Signal 1/1
  FromWs/1 -> Demux/1

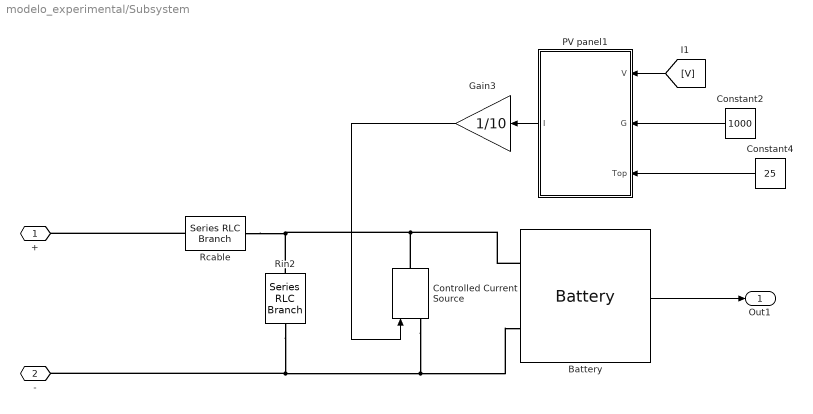
== system modelo_experimental/Subsystem ==
  Battery : electricdrivelib/Extra Sources/Battery  BatType=Lithium-Ion  ShowTempParam=off  ThermalPreset=no  ShowAgeParam=off  NomV=1000  NomQ=20  SOC=100  Batt_Tr=10e-3  PresetModel=off  MaxQ=1  MinV=825  FullV=1280.3859  Dis_rate=200  R=50e-3  Normal_OP=0.90435  expZone="[1188.4244    0.049130435]"  current=[6.5 13 32.5 50]  Units=Time  Tci=20  NomT=20  T2=-30  MaxQ2=4.8  FullV2=7.1  Normal_OP2=5.655  expZone2="[6.58           1]"  Rca=0.6  ti=2000  Dp=0  Neq0=0  Tsim=1e6  Ta1=25  Qeol=5.4*0.9  Reol=0.013333*1.2  Char_age=[2.3478, 3]  Dis_age=[2.3478, 10]  N1=1500  N2=10500  N3=1000  N4=1400  Ta2=45  N5=950
  Constant2 : Constant  Value=1000
  Constant4 : Constant  Value=25
  Controlled Current Source : powerlib/Electrical Sources/Controlled Current Source  Initialize=on  Source_Type=AC  Amplitude=0  Phase=0  Frequency=0  Measurements=None
  Gain3 : Gain  Gain=1/10
  PV panel1 : Subsystem
      mask Display: image('panel.jpg')
  Rcable : powerlib/Elements/Series RLC Branch  LConnTagsString=__new0  RConnTagsString=__new0  BranchType=R  Resistance=1e-3  Inductance=1e-3  SetiL0=off  InitialCurrent=0  Capacitance=1e-6  Setx0=off  InitialVoltage=0  Measurements=None
  Rin2 : powerlib/Elements/Series RLC Branch  LConnTagsString=__new0  RConnTagsString=__new0  BranchType=C  Resistance=.001  Inductance=0  SetiL0=off  InitialCurrent=0  Capacitance=1000e-6  Setx0=off  InitialVoltage=0  Measurements=None
  + : PMIOPort  Side=Left
  - : PMIOPort  Port=2  Side=Left
  Out1 : Outport
  wires:
  PV panel1/1(I) -> Gain3/1
  Gain3/1 -> Controlled Current Source/1
  Battery/1 -> Out1/1
  Constant4/1 -> PV panel1/3(Top)
  Constant2/1 -> PV panel1/2(G)
  [V] -> PV panel1/1(V)
  connections:
  Rcable/RConn1 -- +/RConn1
  Battery/LConn1 -- Controlled Current Source/RConn1 -- Rcable/LConn1 -- Rin2/LConn1
  Battery/LConn2 -- -/RConn1 -- Rin2/RConn1 -- Controlled Current Source/LConn1

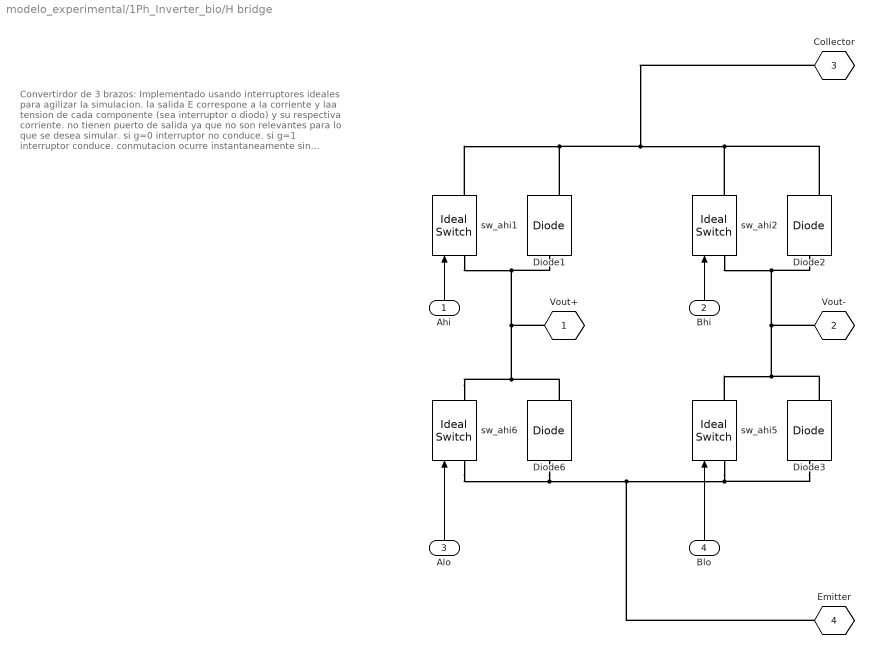
== system modelo_experimental/1Ph_Inverter_bio/H bridge ==
  note: Convertirdor de 3 brazos:
      |
      | Implementado usando interruptores
      | ideales para agilizar la simulacion.
      | la salida E correspone a la corriente y laa
      | tension de cada componente
      | (sea interruptor o diodo) y su respectiva
      | corriente. no tienen puerto de salida ya que no
      | son relevantes para lo que se desea simular.
      |
      | si g=0 interruptor no conduce.
      | si g=1 interruptor conduce.
      |
      | conmutacion ocurre instantaneamente sin
      | retardo.
  Ahi : Inport
  Bhi : Inport  Port=2
  Alo : Inport  Port=3
  Blo : Inport  Port=4
   sw_ahi{1..2,5..6} (4 alike) : powerlib/Power Electronics/Ideal Switch  Ron=0.1  Lon=0  IC=0  Rs=1e6  Cs=10e-12  Measurements=on
  Diode{1..3,6} (4 alike) : powerlib/Power Electronics/Diode  Ron=.2  Lon=0  Vf=0.8  IC=0  UseSnubber=0  Rs=0  Cs=0  Measurements=on
  " Vout+" : PMIOPort  Tag=PMCPort  Side=Right
  Vout- : PMIOPort  Tag=PMCPort  Port=2  Side=Right
  Collector : PMIOPort  Tag=PMCPort  Port=3  Side=Right
  Emitter : PMIOPort  Tag=PMCPort  Port=4  Side=Right
  wires:
  Alo/1 -> " sw_ahi6"/1
  Ahi/1 -> " sw_ahi1"/1
  Blo/1 -> " sw_ahi5"/1
  Bhi/1 -> " sw_ahi2"/1
  connections:
  Diode3/RConn1 -- Vout-/RConn1 -- " sw_ahi2"/LConn1 -- Diode2/LConn1 -- " sw_ahi5"/RConn1
  Diode3/LConn1 -- Emitter/RConn1 -- Diode6/LConn1 -- " sw_ahi6"/LConn1 -- " sw_ahi5"/LConn1
  Diode2/RConn1 -- Collector/RConn1 -- " sw_ahi1"/RConn1 -- Diode1/RConn1 -- " sw_ahi2"/RConn1
  " sw_ahi6"/RConn1 -- Diode6/RConn1 -- " Vout+"/RConn1 -- Diode1/LConn1 -- " sw_ahi1"/LConn1

== system modelo_experimental/1Ph_Inverter_bio/Io_measure ==
  A_current : Inport
  Enable : EnablePort
  Hw1 : dsparch4/Analog Filter Design  method=Bessel  filttype=Lowpass  N=2  Wlo=7000*2*pi  Whi=80  Rp=2  Rs=80
  Transfer Fcn : TransferFcn  Denominator=[1e-6 1]
  Out1 : Outport
  wires:
  Transfer Fcn/1 -> Hw1/1
  A_current/1 -> Transfer Fcn/1
  Hw1/1 -> Out1/1

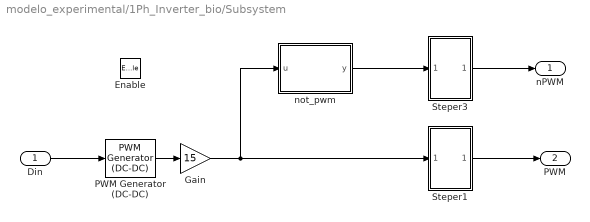
== system modelo_experimental/1Ph_Inverter_bio/Subsystem ==
  Din : Inport
  Enable : EnablePort
  Gain : Gain  Gain=15
  PWM Generator (DC-DC) : powerlib_meascontrol/Pulse & Signal Generators/PWM Generator (DC-DC)  Fsw=f_sw  Ts=samp_f
  Steper1 : Subsystem
  Steper3 : Subsystem
  not_pwm : MATLAB Function  TreatAsAtomicUnit=on
  nPWM : Outport
  PWM : Outport  Port=2
  wires:
  not_pwm/1(y) -> Steper3/1(In1)
  Steper3/1(Out1) -> nPWM/1
  Gain/1 -> Steper1/1(In1), not_pwm/1(u)
  Din/1 -> PWM Generator (DC-DC)/1
  PWM Generator (DC-DC)/1 -> Gain/1
  Steper1/1(Out1) -> PWM/1

== system modelo_experimental/1Ph_Inverter_bio/Subsystem1 ==
  A_volts : Inport
  Enable : EnablePort
  Hw4 : dsparch4/Analog Filter Design  method=Bessel  filttype=Lowpass  N=2  Wlo=7000*2*pi  Whi=80  Rp=2  Rs=80
  Transfer Fcn1 : TransferFcn  Denominator=[1e-6 1]
  Out1 : Outport
  wires:
  A_volts/1 -> Transfer Fcn1/1
  Transfer Fcn1/1 -> Hw4/1
  Hw4/1 -> Out1/1

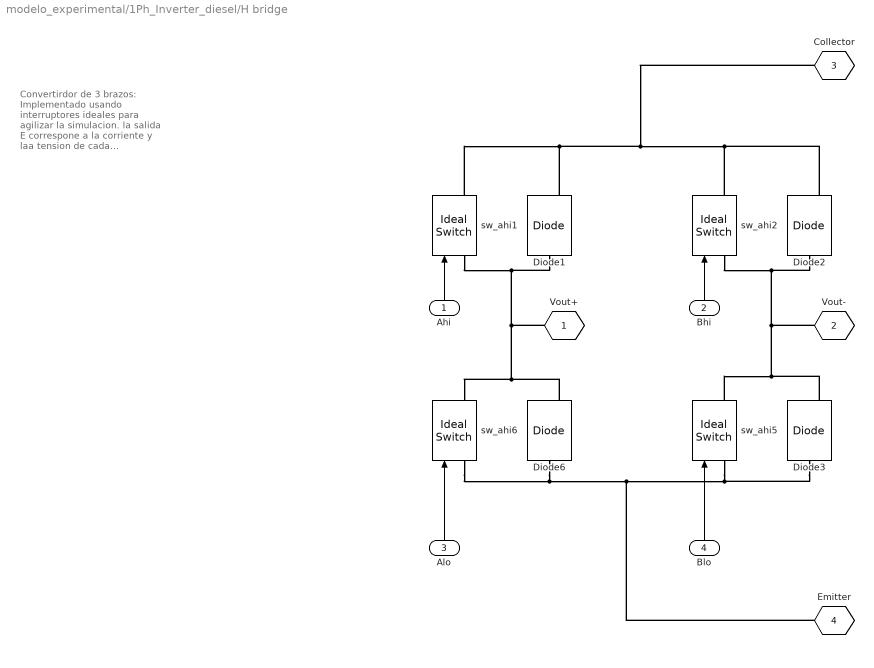
== system modelo_experimental/1Ph_Inverter_diesel/H bridge ==
  note: Convertirdor de 3 brazos:
      |
      | Implementado usando interruptores
      | ideales para agilizar la simulacion.
      | la salida E correspone a la corriente y laa
      | tension de cada componente
      | (sea interruptor o diodo) y su respectiva
      | corriente. no tienen puerto de salida ya que no
      | son relevantes para lo que se desea simular.
      |
      | si g=0 interruptor no conduce.
      | si g=1 interruptor conduce.
      |
      | conmutacion ocurre instantaneamente sin
      | retardo.
  Ahi : Inport
  Bhi : Inport  Port=2
  Alo : Inport  Port=3
  Blo : Inport  Port=4
   sw_ahi{1..2,5..6} (4 alike) : powerlib/Power Electronics/Ideal Switch  Ron=0.1  Lon=0  IC=0  Rs=1e6  Cs=10e-12  Measurements=on
  Diode{1..3,6} (4 alike) : powerlib/Power Electronics/Diode  Ron=.2  Lon=0  Vf=0.8  IC=0  UseSnubber=0  Rs=0  Cs=0  Measurements=on
  " Vout+" : PMIOPort  Tag=PMCPort  Side=Right
  Vout- : PMIOPort  Tag=PMCPort  Port=2  Side=Right
  Collector : PMIOPort  Tag=PMCPort  Port=3  Side=Right
  Emitter : PMIOPort  Tag=PMCPort  Port=4  Side=Right
  wires:
  Bhi/1 -> " sw_ahi2"/1
  Blo/1 -> " sw_ahi5"/1
  Ahi/1 -> " sw_ahi1"/1
  Alo/1 -> " sw_ahi6"/1
  connections:
  " sw_ahi1"/LConn1 -- Diode1/LConn1 -- " Vout+"/RConn1 -- Diode6/RConn1 -- " sw_ahi6"/RConn1
  " sw_ahi2"/RConn1 -- Diode1/RConn1 -- " sw_ahi1"/RConn1 -- Collector/RConn1 -- Diode2/RConn1
  " sw_ahi5"/LConn1 -- " sw_ahi6"/LConn1 -- Diode6/LConn1 -- Emitter/RConn1 -- Diode3/LConn1
  " sw_ahi5"/RConn1 -- Diode2/LConn1 -- " sw_ahi2"/LConn1 -- Vout-/RConn1 -- Diode3/RConn1

== system modelo_experimental/1Ph_Inverter_diesel/Io_measure ==
  A_current : Inport
  Enable : EnablePort
  Hw7 : dsparch4/Analog Filter Design  method=Bessel  filttype=Lowpass  N=2  Wlo=7000*2*pi  Whi=80  Rp=2  Rs=80
  Transfer Fcn : TransferFcn  Denominator=[1e-6 1]
  Out1 : Outport
  wires:
  Hw7/1 -> Out1/1
  Transfer Fcn/1 -> Hw7/1
  A_current/1 -> Transfer Fcn/1

== system modelo_experimental/1Ph_Inverter_diesel/Subsystem ==
  Din : Inport
  Enable : EnablePort
  Gain : Gain  Gain=15
  PWM Generator (DC-DC) : powerlib_meascontrol/Pulse & Signal Generators/PWM Generator (DC-DC)  Fsw=f_sw  Ts=samp_f
  Steper1 : Subsystem
  Steper3 : Subsystem
  not_pwm : MATLAB Function  TreatAsAtomicUnit=on
  nPWM : Outport
  PWM : Outport  Port=2
  wires:
  PWM Generator (DC-DC)/1 -> Gain/1
  Gain/1 -> not_pwm/1(u), Steper1/1(In1)
  Din/1 -> PWM Generator (DC-DC)/1
  not_pwm/1(y) -> Steper3/1(In1)
  Steper3/1(Out1) -> nPWM/1
  Steper1/1(Out1) -> PWM/1

== system modelo_experimental/1Ph_Inverter_diesel/Vo_measure ==
  A_volts : Inport
  Enable : EnablePort
  Hw3 : dsparch4/Analog Filter Design  method=Bessel  filttype=Lowpass  N=2  Wlo=7000*2*pi  Whi=80  Rp=2  Rs=80
  Transfer Fcn1 : TransferFcn  Denominator=[1e-6 1]
  Out1 : Outport
  wires:
  Transfer Fcn1/1 -> Hw3/1
  Hw3/1 -> Out1/1
  A_volts/1 -> Transfer Fcn1/1

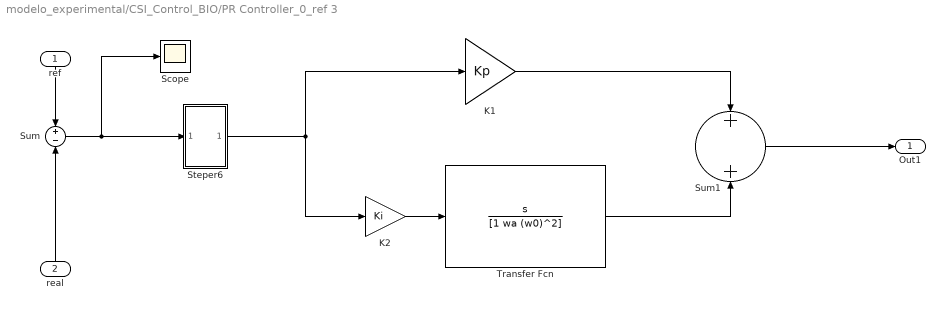
== system modelo_experimental/CSI_Control_BIO/PR Controller_0_ref 3 ==
  ref : Inport
  real : Inport  Port=2
  K1 : Gain  Gain=Kp
  K2 : Gain  Gain=Ki
  Scope : Scope
  Steper6 : Subsystem
  Sum : Sum  Inputs=+-
  Sum1 : Sum  Inputs=+|+
  Transfer Fcn : TransferFcn  Numerator=[1 0]  Denominator=[1 wa (w0)^2]
  Out1 : Outport
  wires:
  real/1 -> Sum/2
  ref/1 -> Sum/1
  Sum/1 -> Scope/1, Steper6/1(In1)
  K1/1 -> Sum1/1
  Transfer Fcn/1 -> Sum1/2
  K2/1 -> Transfer Fcn/1
  Steper6/1(Out1) -> K1/1, K2/1
  Sum1/1 -> Out1/1

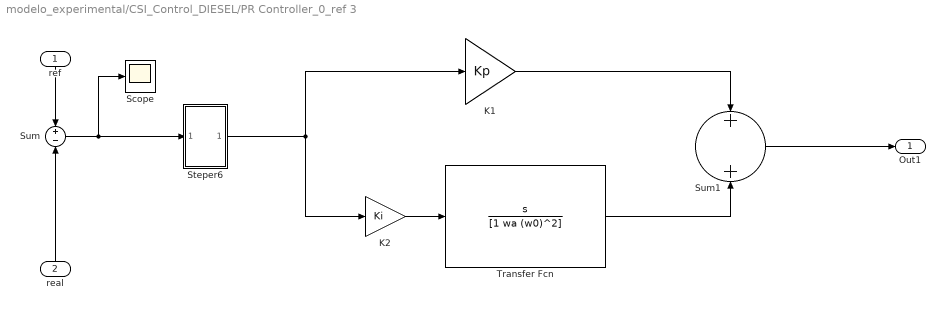
== system modelo_experimental/CSI_Control_DIESEL/PR Controller_0_ref 3 ==
  ref : Inport
  real : Inport  Port=2
  K1 : Gain  Gain=Kp
  K2 : Gain  Gain=Ki
  Scope : Scope
  Steper6 : Subsystem
  Sum : Sum  Inputs=+-
  Sum1 : Sum  Inputs=+|+
  Transfer Fcn : TransferFcn  Numerator=[1 0]  Denominator=[1 wa (w0)^2]
  Out1 : Outport
  wires:
  Sum1/1 -> Out1/1
  Steper6/1(Out1) -> K2/1, K1/1
  K2/1 -> Transfer Fcn/1
  Transfer Fcn/1 -> Sum1/2
  K1/1 -> Sum1/1
  Sum/1 -> Scope/1, Steper6/1(In1)
  ref/1 -> Sum/1
  real/1 -> Sum/2

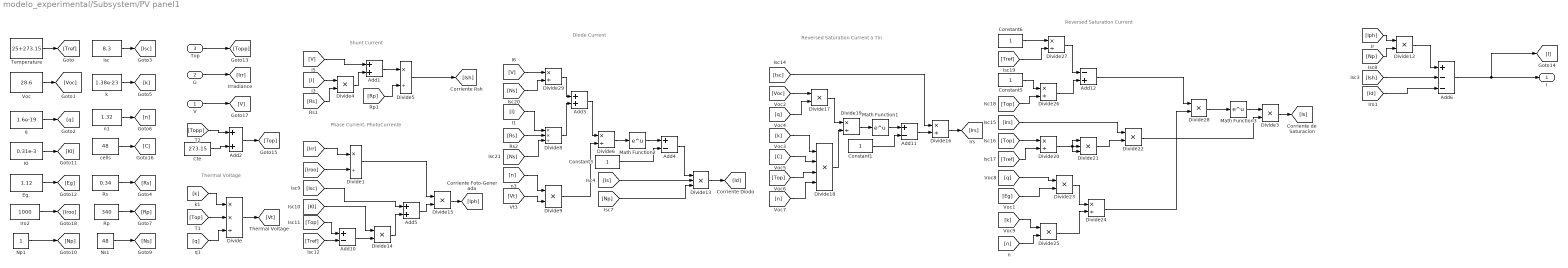
== system modelo_experimental/Subsystem/PV panel1 ==
  note: Thermal Voltage
  note: Shunt Current
  note: Phase Current- PhotoCurrente
  note: Diode Current
  note: Reversed Saturation Current a Tin
  note: Reversed Saturation Current
  V : Inport
  G : Inport  Port=2
  Top : Inport  Port=3
  Add{1..3,5} (4 alike) : Sum
  Add10 : Sum  Inputs=+-
  Add11 : Sum  Inputs=+-
  Add12 : Sum  Inputs=-+
  Add4 : Sum  Inputs=+-
  Add6 : Sum  Inputs=+--
  Constant{1,3,5..6} (4 alike) : Constant
  Cte : Constant  Value=273.15
  Divide : Product  Inputs=**/
  Divide{1,5..6,16,19..20,24,26..27,29} (10 alike) : Product  Inputs=*/
  Divide{3..4,9,12,14..15,17,22..23,25,28} (11 alike) : Product  Inputs=**
  Divide13 : Product  Inputs=***
  Divide18 : Product  Inputs=****
  Divide21 : Product  Inputs=***
  Divide8 : Product  Inputs=**/
  Eg. : Constant  Value=1.12
  Iro2 : Constant  Value=1000
  Isc : Constant  Value=8.3
  KI : Constant  Value=0.31e-3
  Math Function1 : Math  SaturateOnIntegerOverflow=on
  Math Function2 : Math  SaturateOnIntegerOverflow=on
  Math Function3 : Math  SaturateOnIntegerOverflow=on
  Np1 : Constant
  Ns1 : Constant  Value=48
  Rp : Constant  Value=340
  Rs : Constant  Value=0.34
  Temperature : Constant  Value=25+273.15
  Voc : Constant  Value=28.6
  cells : Constant  Value=48
  k : Constant  Value=1.38e-23
  n1 : Constant  Value=1.32
  q : Constant  Value=1.6e-19
  I : Outport
  wires:
  Temperature/1 -> [Tref]
  Voc/1 -> [Voc]
  q/1 -> [q]
  Isc/1 -> [Isc]
  k/1 -> [k]
  n1/1 -> [n]
  [k] -> Divide/1
  [Top] -> Divide/2
  [q] -> Divide/3
  Divide/1 -> [Vt]
  Divide3/1 -> [Is]
  [Ish] -> Add6/2
  Add6/1 -> I/1, [I]
  [I] -> Divide8/1
  [Rs] -> Divide8/2
  Divide8/1 -> Add3/2
  [n] -> Divide9/1
  [Vt] -> Divide9/2
  Divide9/1 -> Divide6/2
  Add3/1 -> Divide6/1
  Divide6/1 -> Math Function2/1
  Math Function2/1 -> Add4/1
  Add4/1 -> Divide13/1
  [Is] -> Divide13/2
  Divide13/1 -> [Id]
  Divide4/1 -> Add1/2
  Add1/1 -> Divide5/1
  [Rp] -> Divide5/2
  Divide5/1 -> [Ish]
  [Rs] -> Divide4/2
  [I] -> Divide4/1
  KI/1 -> [KI]
  Eg./1 -> [Eg]
  [V] -> Add1/1
  [Np] -> Divide13/3
  [Iph] -> Divide12/1
  [Np] -> Divide12/2
  Divide12/1 -> Add6/1
  [Isc] -> Add5/1
  [Top] -> Add10/1
  [Tref] -> Add10/2
  Add10/1 -> Divide14/2
  [KI] -> Divide14/1
  [Voc] -> Divide17/1
  [q] -> Divide17/2
  [k] -> Divide18/1
  [C] -> Divide18/2
  [Top] -> Divide18/3
  [n] -> Divide18/4
  Divide17/1 -> Divide19/1
  Divide18/1 -> Divide19/2
  Divide19/1 -> Math Function1/1
  Constant1/1 -> Add11/2
  Math Function1/1 -> Add11/1
  Add11/1 -> Divide16/2
  Divide16/1 -> [Irs]
  [Tref] -> Divide20/2
  [Top] -> Divide20/1
  Divide20/1 -> Divide21/2, Divide21/1, Divide21/3
  Divide21/1 -> Divide22/2
  [Irs] -> Divide22/1
  [q] -> Divide23/1
  Divide23/1 -> Divide24/1
  [k] -> Divide25/1
  [n] -> Divide25/2
  Divide25/1 -> Divide24/2
  Constant5/1 -> Divide26/1
  [Top] -> Divide26/2
  Constant6/1 -> Divide27/1
  [Tref] -> Divide27/2
  Divide27/1 -> Add12/1
  Divide26/1 -> Add12/2
  Add12/1 -> Divide28/1
  Divide24/1 -> Divide28/2
  Divide28/1 -> Math Function3/1
  Divide29/1 -> Add3/1
  [Ns] -> Divide29/2
  [V] -> Divide29/1
  [Ns] -> Divide8/3
  Divide14/1 -> Add5/2
  Add5/1 -> Divide15/2
  Divide15/1 -> [Iph]
  V/1 -> [V]
  G/1 -> [Irr]
  Top/1 -> [Topp]
  cells/1 -> [C]
  [Id] -> Add6/3
  Cte/1 -> Add2/2
  Add2/1 -> [Top]
  [Topp] -> Add2/1
  [Irr] -> Divide1/1
  [Iroo] -> Divide1/2
  Divide1/1 -> Divide15/1
  Iro2/1 -> [Iroo]
  Rs/1 -> [Rs]
  Rp/1 -> [Rp]
  Ns1/1 -> [Ns]
  Np1/1 -> [Np]
  Constant3/1 -> Add4/2
  [Isc] -> Divide16/1
  Math Function3/1 -> Divide3/1
  Divide22/1 -> Divide3/2
  [Eg] -> Divide23/2

== system modelo_experimental/1Ph_Inverter_bio/Subsystem/Steper1 ==
  In1 : Inport
  Product : Product
  Step : Step  Time=st_time  SampleTime=samp_f
  Out1 : Outport
  wires:
  Step/1 -> Product/2
  In1/1 -> Product/1
  Product/1 -> Out1/1

== system modelo_experimental/1Ph_Inverter_bio/Subsystem/Steper3 ==
  In1 : Inport
  Product : Product
  Step : Step  Time=st_time  SampleTime=samp_f
  Out1 : Outport
  wires:
  Product/1 -> Out1/1
  In1/1 -> Product/1
  Step/1 -> Product/2

== system modelo_experimental/1Ph_Inverter_diesel/Subsystem/Steper1 ==
  In1 : Inport
  Product : Product
  Step : Step  Time=st_time  SampleTime=samp_f
  Out1 : Outport
  wires:
  Product/1 -> Out1/1
  In1/1 -> Product/1
  Step/1 -> Product/2

== system modelo_experimental/1Ph_Inverter_diesel/Subsystem/Steper3 ==
  In1 : Inport
  Product : Product
  Step : Step  Time=st_time  SampleTime=samp_f
  Out1 : Outport
  wires:
  Step/1 -> Product/2
  In1/1 -> Product/1
  Product/1 -> Out1/1

== system modelo_experimental/CSI_Control_BIO/PR Controller_0_ref 3/Steper6 ==
  In1 : Inport
  Product : Product
  Step : Step  Time=st_time  SampleTime=0
  Out1 : Outport
  wires:
  Product/1 -> Out1/1
  In1/1 -> Product/1
  Step/1 -> Product/2

== system modelo_experimental/CSI_Control_DIESEL/PR Controller_0_ref 3/Steper6 ==
  In1 : Inport
  Product : Product
  Step : Step  Time=st_time  SampleTime=0
  Out1 : Outport
  wires:
  Step/1 -> Product/2
  In1/1 -> Product/1
  Product/1 -> Out1/1

== matlab function modelo_experimental/1Ph_Inverter_diesel/Subsystem/not_pwm ==
  data: u input; y output
function y = fcn(u)
%#codegen

if(u==0 || u<0)
    a=15;
else
    a=0;
end;

y = a;

== matlab function modelo_experimental/1Ph_Inverter_bio/Subsystem/not_pwm ==
  data: u input; y output
function y = fcn(u)
%#codegen

if(u==0 || u<0)
    a=15;
else
    a=0;
end;

y = a;

== matlab function modelo_experimental/CSI_Control_BIO/PQ_singlePhase ==
  data: va input; p output; vb input; ia input; ib input; q output
function [p, q] = fcn(va, vb, ia, ib)
% Esta funcion calcula la potencia activa y reactiva instantanea
% para el caso mnosofasico. En la revision de 2 papers he observado
% que una manera de extender la teoria de potencia al caso monofasico
% es asumiendo la tension o corriente de una fase como la componente
% alpha y hacer un desfase de 90 grados para obtener una version
% artificial de beta.

paux=va*ia+vb*ib;
if(paux > 20e4)
    paux = 20e4;
end
if(paux < -20e4)
    paux = -20e-4;
end

p = paux/2; % potencia activa instantanea

qaux = vb*ia-va*ib;

if(qaux>20e4)
    qaux=20e4;
end
if(qaux<-20e4)
    qaux=-20e4;
end

q = qaux/2; % potencia reactiva instantanea

== matlab function modelo_experimental/CSI_Control_DIESEL/PQ2AlphBetaCurrents_SinglePhase ==
  data: Va input; Ia output; Vb input; p input; q input; Ib output
function [Ia, Ib] = fcn(Va, Vb, p, q)
%#codegen

% divide by zero protection
if(abs((Va^2+Vb^2))<=1000*eps(0))
    det = 1/eps(0);
else
    det = 1/(Va^2+Vb^2); % constante auxiliar
end;
%det = 1/(Va^2+Vb^2);

Mat = det*[Va Vb; Vb -Va];
Iab = Mat*[2*p;2*q];

Iaaux = Iab(1);
Ibaux = Iab(2);

ilim=1e3;

if(Iaaux>ilim)
    Iaaux=ilim;
end;
if(Iaaux<-ilim)
    Iaaux =-ilim;    
end;

if(isnan(Iaaux))
    Iaaux=0;
end;
%-----------------


if(Ibaux>ilim)
    Ibaux=ilim;
end;
if(Ibaux<-ilim)
    Ibaux =-ilim;    
end;

if(isnan(Ibaux))
    Ibaux=0;
end;
%-----------------


Ia = Iaaux;
Ib = Ibaux;

== matlab function modelo_experimental/CSI_Control_DIESEL/PQ_singlePhase ==
  data: va input; p output; vb input; ia input; ib input; q output
function [p, q] = fcn(va, vb, ia, ib)
% Esta funcion calcula la potencia activa y reactiva instantanea
% para el caso mnosofasico. En la revision de 2 papers he observado
% que una manera de extender la teoria de potencia al caso monofasico
% es asumiendo la tension o corriente de una fase como la componente
% alpha y hacer un desfase de 90 grados para obtener una version
% artificial de beta.

paux=va*ia+vb*ib;
if(paux > 20e4)
    paux = 20e4;
end
if(paux < -20e4)
    paux = -20e-4;
end

p = paux/2; % potencia activa instantanea

qaux = vb*ia-va*ib;

if(qaux>20e4)
    qaux=20e4;
end
if(qaux<-20e4)
    qaux=-20e4;
end

q = qaux/2; % potencia reactiva instantanea

== matlab function modelo_experimental/CSI_Control_BIO/PQ2AlphBetaCurrents_SinglePhase ==
  data: Va input; Ia output; Vb input; p input; q input; Ib output
function [Ia, Ib] = fcn(Va, Vb, p, q)
%#codegen

% divide by zero protection
if(abs((Va^2+Vb^2))<=1000*eps(0))
    det = 1/eps(0);
else
    det = 1/(Va^2+Vb^2); % constante auxiliar
end;
%det = 1/(Va^2+Vb^2);

Mat = det*[Va Vb; Vb -Va];
Iab = Mat*[2*p;2*q];

Iaaux = Iab(1);
Ibaux = Iab(2);

ilim=1e3;

if(Iaaux>ilim)
    Iaaux=ilim;
end;
if(Iaaux<-ilim)
    Iaaux =-ilim;    
end;

if(isnan(Iaaux))
    Iaaux=0;
end;
%-----------------


if(Ibaux>ilim)
    Ibaux=ilim;
end;
if(Ibaux<-ilim)
    Ibaux =-ilim;    
end;

if(isnan(Ibaux))
    Ibaux=0;
end;
%-----------------


Ia = Iaaux;
Ib = Ibaux;
